simulink model "a"  (R2018a)
settings: Solver=FixedStepDiscrete  StartTime=0.0  StopTime=10.0  RelTol=1e-3
libraries: dsparch4 x1
settings Model: Creator=salman  LastModifiedBy=salman
settings OptimizationCC: DefaultParameterBehavior=Inlined  UseDivisionForNetSlopeComputation=on  UseFloatMulNetSlope=on  InlineInvariantSignals=on  PassReuseOutputArgsAs=Individual arguments  ZeroExternalMemoryAtStartup=off  ZeroInternalMemoryAtStartup=off  NoFixptDivByZeroProtection=on  EfficientFloat2IntCast=on  LifeSpan=1  OptimizeBlockOrder=speed  DifferentSizesBufferReuse=on
settings DebuggingCC: ParameterTunabilityLossMsg=error
settings HardwareCC: ProdLongLongMode=on
settings SFSimCC: MATLABDynamicMemAlloc=off
settings RTWCC: SystemTargetFile=ert.tlc  TemplateMakefile=ert_default_tmf  GenerateReport=on  IncludeHyperlinkInReport=on  LaunchReport=on  GenerateTraceInfo=on  GenerateTraceReport=on  GenerateTraceReportSl=on  GenerateTraceReportSf=on  GenerateTraceReportEml=on  GenerateCodeMetricsReport=on
settings CodeAppCC: ForceParamTrailComments=on  IgnoreCustomStorageClasses=off  OperatorAnnotations=on  SimulinkDataObjDesc=on  SFDataObjDesc=on  CustomSymbolStrGlobalVar=rt$N$M  CustomSymbolStrType=$N$M  CustomSymbolStrFcn=$N$M$F  CustomSymbolStrMacro=$N$M  InsertBlockDesc=on
settings ERTTargetCC: TargetLangStandard=C99 (ISO)  GenerateSampleERTMain=on  IncludeMdlTerminateFcn=off  CombineSignalStateStructs=on  SuppressErrorStatus=on  SupportComplex=off  InlinedParameterPlacement=NonHierarchical  ERTCustomFileTemplate=example_file_process.tlc  ERTFilePackagingFormat=CompactWithDataFile

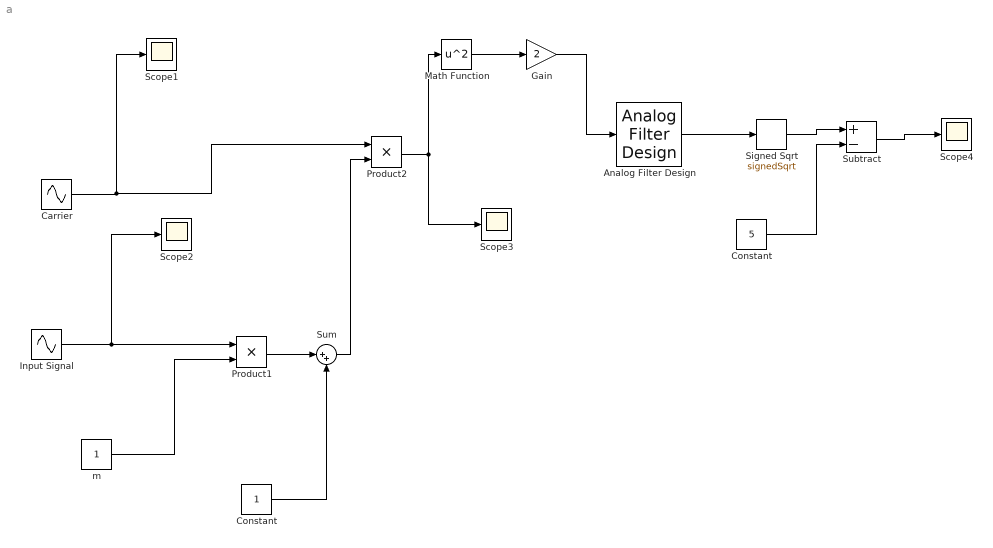
== system a ==
  Analog Filter Design : dsparch4/Analog Filter Design  method=Butterworth  filttype=Lowpass  N=8  Wlo=30  Whi=80  Rp=2  Rs=40
  "Carrier " : Sin  Amplitude=5  Frequency=2*pi*25  SampleTime=1/8000
  Constant : Constant  Value=5
  "Constant " : Constant
  Gain : Gain  Gain=2
  "Input Signal " : Sin  Frequency=2*pi  SampleTime=1/8000
  Math Function : Math  Operator=square  SaturateOnIntegerOverflow=on
  "Product1 " : Product
  "Product2 " : Product
  "Scope1 " : Scope
  "Scope2 " : Scope
  "Scope3 " : Scope
  "Scope4 " : Scope
  Signed Sqrt : Sqrt  Operator=signedSqrt  SaturateOnIntegerOverflow=on
  Subtract : Sum  Inputs=+-
  Sum : Sum  Inputs=|++
  "m " : Constant
  wires:
  "Product2 "/1 -> "Scope3 "/1, Math Function/1
  "Product1 "/1 -> Sum/1
  Sum/1 -> "Product2 "/2
  "m "/1 -> "Product1 "/2
  "Carrier "/1 -> "Product2 "/1, "Scope1 "/1
  "Input Signal "/1 -> "Product1 "/1, "Scope2 "/1
  "Constant "/1 -> Sum/2
  Analog Filter Design/1 -> Signed Sqrt/1
  Subtract/1 -> "Scope4 "/1
  Signed Sqrt/1 -> Subtract/1
  Constant/1 -> Subtract/2
  Math Function/1 -> Gain/1
  Gain/1 -> Analog Filter Design/1
